simulink model "sistemacompleto_LTI_aumentado"  (R2023b)
settings: Solver=VariableStepAuto  StartTime=0.0  StopTime=1  RelTol=1e-3
settings Model: Creator=nahue  LastModifiedBy=nahue

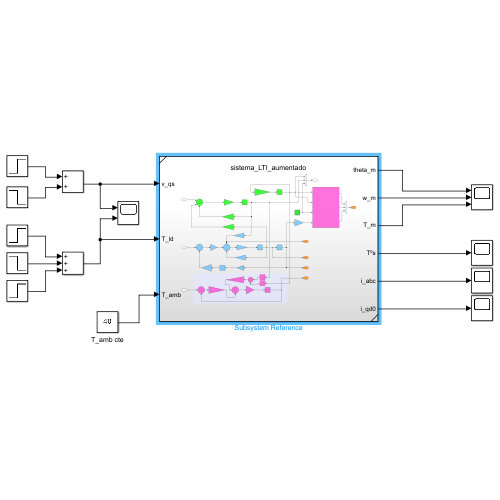
[thumbnail: Simulink's stored preview of the top-level diagram]
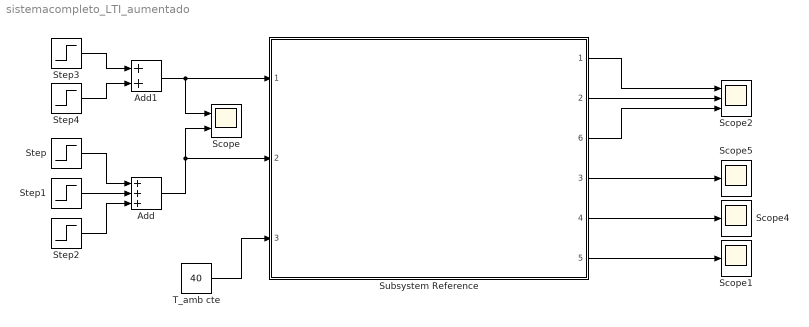
== system sistemacompleto_LTI_aumentado ==
  Add : Sum  Inputs=+++
  Add1 : Sum
  Scope : Scope  NumInputPorts=2
  Scope1 : Scope
  Scope2 : Scope  NumInputPorts=3
  Scope4 : Scope
  Scope5 : Scope
  Step : Step  Time=0.3  After=6.28  SampleTime=0.05
  Step1 : Step  Time=0.5  After=-6.28*2  SampleTime=0.05
  Step2 : Step  Time=0.9  After=6.28  SampleTime=0.05
  Step3 : Step  Time=0.1  After=19.596  SampleTime=0.05
  Step4 : Step  Time=0.7  After=-19.596  SampleTime=0.05
  Subsystem Reference : Subsystem  ReferencedSubsystem=sistema_LTI_aumentado
      settings: PortSchema="{\"entries\":[{\"content\":{\"sides\":[{\"content\":{\"connectorIds\":[\"In1\",\"In2\",\"In3\"]},\"type\":\"ConnectorPlacement.EquallySpacedRectSide\",\"uuid\":\"a9fd203c-ee17-4a6f-9e49-b32a3c269841\"},{\"content\":{\"connectorIds\":[\"Out1\",\"Out2\",\"Out6\",\"Out3\",\"Out4\",\"Out5\"],\"side\":\"RIGHT\"},\"type\":\"ConnectorPlacement.EquallySpacedRectSide\",\"uuid\":\"bfddeaa7-7e9a-4fa0-b9ed-acae47f219cd\"},{\"content\":{\"side\":\"TOP\"},\"type\":\"ConnectorPlacement.EquallySpacedRectSide\",\"uuid\":\"01d68b23-e98f-4920-a18d-a9ccf9d9987a\"}]},\"type\":\"ConnectorPlacement.EquallySpacedConnector\",\"uuid\":\"92ceb62a-c405-4175-b2fa-7bbb7bcd3818\"}],\"packageUris\":[\"http://schema.mathworks.com/mf0/Connector/R2020b\"],\"version\":\"1.0\"}"
  T_amb cte : Constant  Value=40
  wires:
  Step3/1 -> Add1/1
  Step/1 -> Add/1
  Step1/1 -> Add/2
  Add1/1 -> Scope/1, Subsystem Reference/1
  Step2/1 -> Add/3
  Add/1 -> Scope/2, Subsystem Reference/2
  Step4/1 -> Add1/2
  T_amb cte/1 -> Subsystem Reference/3
  Subsystem Reference/4 -> Scope4/1
  Subsystem Reference/5 -> Scope1/1
  Subsystem Reference/1 -> Scope2/1
  Subsystem Reference/2 -> Scope2/2
  Subsystem Reference/6 -> Scope2/3
  Subsystem Reference/3 -> Scope5/1
